simulink model "feedback_lin"  (R2022b)
settings: Solver=ode4  StartTime=0.0  StopTime=t_end  FixedStep=t_step  RelTol=1e-3
undefined symbols (not defined in the file): AW, C, d_delta, d_on, d_time, d_val, E, iL0, K0i, K1i, K_r, Ki, Kif, Kn, Kti, Ku, L, n_on, R, r_delta, r_on, r_sel, r_time, r_val, sel, sigma_n, t_step, uC0, wp, y0
libraries: fuzblock x1
settings Model: Creator=Milosh Yokich  LastModifiedBy=Milosh Yokich
settings SolverCC: AlgebraicLoopSolver=TrustRegion
settings DataIOCC: ReturnWorkspaceOutputs=off
settings DebuggingCC: UnconnectedInputMsg=warning  UnconnectedOutputMsg=warning  UnconnectedLineMsg=warning  SFMachineParentedDataDiag=warning  ArithmeticOperatorsInVariantConditions=warning
settings ModelReferenceCC: EnableRefExpFcnMdlSchedulingChecks=on
settings SFSimCC: SimUseLocalCustomCode=off  CustomCodeUndefinedFunction=UseInterfaceOnly
settings RTWCC: RTWUseLocalCustomCode=off

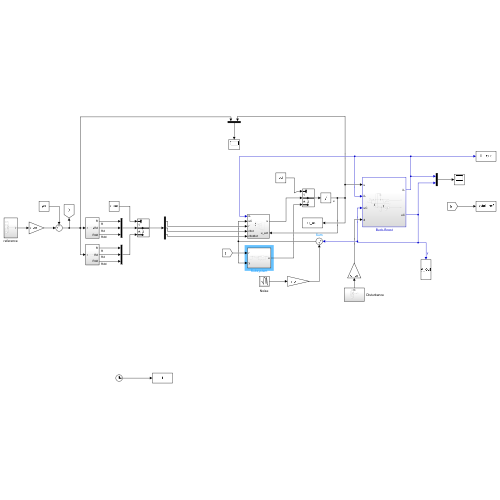
[thumbnail: Simulink's stored preview of the top-level diagram]
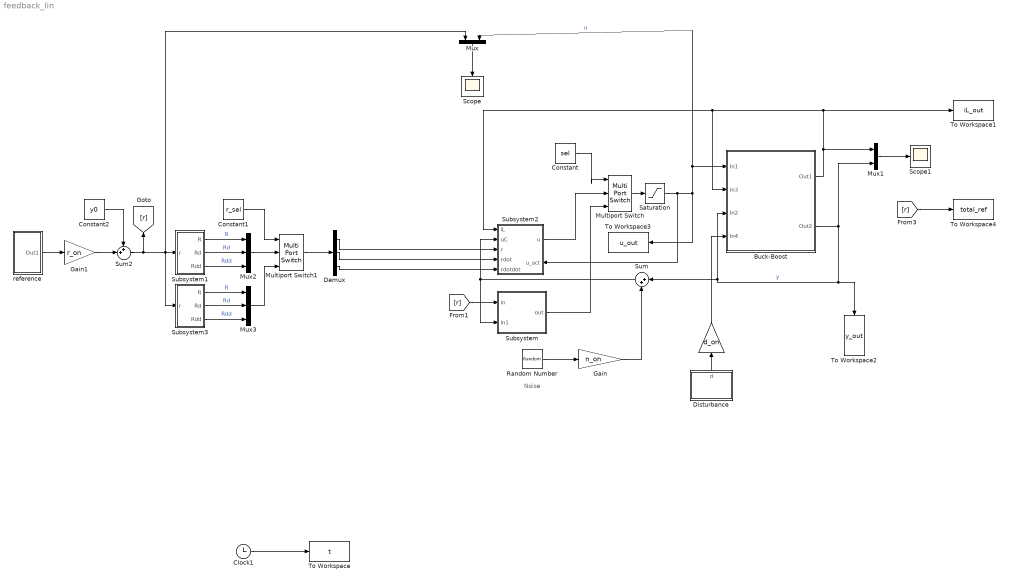
== system feedback_lin ==
  note: Noise
  " " : Gain  Gain=d_on
  Buck-Boost : Subsystem
  Clock1 : Clock
  Constant : Constant  Value=sel
  Constant1 : Constant  Value=r_sel
  Constant2 : Constant  Value=y0
  Demux : Demux  Outputs=3
  Disturbance : Subsystem
  Gain : Gain  Gain=n_on
  Gain1 : Gain  Gain=r_on
  Multiport Switch : MultiPortSwitch  Inputs=2  SaturateOnIntegerOverflow=off  InputSameDT=off
  Multiport Switch1 : MultiPortSwitch  Inputs=2  SaturateOnIntegerOverflow=off  InputSameDT=off
  Mux : Mux  Inputs=2
  Mux1 : Mux  Inputs=2
  Mux2 : Mux  Inputs=3
  Mux3 : Mux  Inputs=3
  Random Number : RandomNumber  Variance=sigma_n  SampleTime=t_step
  Saturation : Saturate  UpperLimit=1  LowerLimit=0
  Scope : Scope
  Scope1 : Scope
  Subsystem : Subsystem
  Subsystem1 : Subsystem
  Subsystem2 : Subsystem
      settings: PortSchema="{\"entries\":[{\"content\":{\"sides\":[{\"content\":{\"connectorIds\":[\"In1\",\"In2\",\"In3\",\"In4\",\"In5\"]},\"type\":\"ConnectorPlacement.EquallySpacedRectSide\",\"uuid\":\"a5ffe97d-c71e-4de0-ba63-bc76db2e4a28\"},{\"content\":{\"connectorIds\":[\"Out1\",\"In6\"],\"side\":\"RIGHT\"},\"type\":\"ConnectorPlacement.EquallySpacedRectSide\",\"uuid\":\"4d46e151-a221-479a-a7c8-fb4e18a057b4\"},{\"content\":{\"connectorIds\":[],\"side\":\"TOP\"},\"type\":\"ConnectorPlacement.EquallySpacedRectSide\",\"uuid\":\"a0b468b3-16b9-437b-958e-968171817142\"},{\"content\":{\"connectorIds\":[],\"side\":\"BOTTOM\"},\"type\":\"ConnectorPlacement.EquallySpacedRectSide\",\"uuid\":\"210b4f3c-ba38-4a79-8d72-0619259306c1\"}]},\"type\":\"ConnectorPlacement.EquallySpacedConnector\",\"uuid\":\"c6942702-5a6a-49ce-9e2c-c5f8d8595752\"}],\"packageUris\":[\"http://schema.mathworks.com/mf0/Connector/R2020b\"],\"version\":\"1.0\"}"
  Subsystem3 : Subsystem
  Sum : Sum  Inputs=|++
  Sum2 : Sum  Inputs=++|
  To Workspace : ToWorkspace  VariableName=t  SampleTime=-1
  To Workspace1 : ToWorkspace  VariableName=iL_out  SampleTime=-1
  To Workspace2 : ToWorkspace  VariableName=y_out  SampleTime=-1
  To Workspace3 : ToWorkspace  VariableName=u_out  SampleTime=-1
  To Workspace4 : ToWorkspace  VariableName=total_ref  SampleTime=-1
  "reference " : Subsystem
  wires:
  Random Number/1 -> Gain/1
  Clock1/1 -> To Workspace/1
  Mux/1 -> Scope/1
  Mux1/1 -> Scope1/1
  Saturation/1 -> Subsystem2/6(u_act), Buck-Boost/1(In1), Mux/2, To Workspace3/1  "u"
  [r] -> To Workspace4/1
  Disturbance/1(d) -> " "/1
  "reference "/1(Out1) -> Gain1/1
  Gain/1 -> Sum/2
  Buck-Boost/2(Out2) -> Buck-Boost/3(In2), Sum/1, To Workspace2/1, Mux1/2  "y"
  Buck-Boost/1(Out1) -> Subsystem2/1(iL), Buck-Boost/2(In3), To Workspace1/1, Mux1/1
  " "/1 -> Buck-Boost/4(In4)
  Constant2/1 -> Sum2/1
  Multiport Switch/1 -> Saturation/1
  Constant/1 -> Multiport Switch/1
  Sum2/1 -> Subsystem3/1(r), Subsystem1/1(r), Mux/1, [r]
  Gain1/1 -> Sum2/2
  Subsystem1/1(R) -> Mux2/1  "R"
  Subsystem1/2(Rd) -> Mux2/2  "Rd"
  Subsystem1/3(Rdd) -> Mux2/3  "Rdd"
  Subsystem3/1(R) -> Mux3/1  "R"
  Subsystem3/2(Rd) -> Mux3/2  "Rd"
  Subsystem3/3(Rdd) -> Mux3/3  "Rdd"
  Mux2/1 -> Multiport Switch1/2
  Mux3/1 -> Multiport Switch1/3
  Constant1/1 -> Multiport Switch1/1
  Multiport Switch1/1 -> Demux/1
  Demux/3 -> Subsystem2/5(rdotdot)
  Demux/2 -> Subsystem2/4(rdot)
  Demux/1 -> Subsystem2/3(r)
  [r] -> Subsystem/1(in)
  Sum/1 -> Subsystem/2(in1), Subsystem2/2(uC)
  Subsystem2/1(u) -> Multiport Switch/2
  Subsystem/1(out) -> Multiport Switch/3

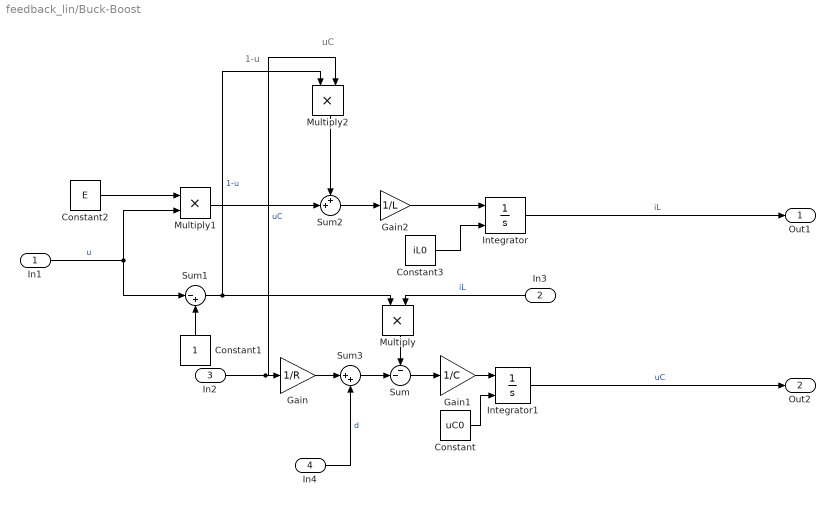
== system feedback_lin/Buck-Boost ==
  note: uC
  note: 1-u
  In1 : Inport
  In3 : Inport  Port=2
  In2 : Inport  Port=3
  In4 : Inport  Port=4
  Constant : Constant  Value=uC0
  Constant1 : Constant
  Constant2 : Constant  Value=E
  Constant3 : Constant  Value=iL0
  Gain : Gain  Gain=1/R
  Gain1 : Gain  Gain=1/C
  Gain2 : Gain  Gain=1/L
  Integrator : Integrator  InitialConditionSource=external
  Integrator1 : Integrator  InitialConditionSource=external
  Multiply : Product
  Multiply1 : Product
  Multiply2 : Product
  Sum : Sum  Inputs=--|
  Sum1 : Sum  Inputs=|-+
  Sum2 : Sum  Inputs=++|
  Sum3 : Sum  Inputs=|++
  Out1 : Outport  VectorParamsAs1DForOutWhenUnconnected=off
  Out2 : Outport  Port=2  VectorParamsAs1DForOutWhenUnconnected=off
  wires:
  In4/1 -> Sum3/2  "d"
  Sum3/1 -> Sum/2
  Gain/1 -> Sum3/1
  In3/1 -> Multiply/2  "iL"
  In2/1 -> Gain/1, Multiply2/2  "uC"
  Sum2/1 -> Gain2/1
  Sum/1 -> Gain1/1
  Constant/1 -> Integrator1/2
  Constant1/1 -> Sum1/2
  Multiply/1 -> Sum/1
  Constant3/1 -> Integrator/2
  In1/1 -> Sum1/1, Multiply1/2  "u"
  Multiply1/1 -> Sum2/2
  Gain1/1 -> Integrator1/1
  Integrator/1 -> Out1/1  "iL"
  Gain2/1 -> Integrator/1
  Sum1/1 -> Multiply2/1, Multiply/1  "1-u"
  Integrator1/1 -> Out2/1  "uC"
  Constant2/1 -> Multiply1/1
  Multiply2/1 -> Sum2/1

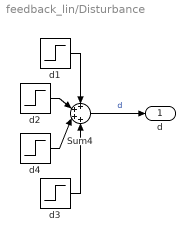
== system feedback_lin/Disturbance ==
  Sum4 : Sum  Inputs=++++
  "d1 " : Step  Time=d_time  After=d_val  SampleTime=0
  "d2 " : Step  Time=d_time + d_delta  After=-d_val  SampleTime=0
  "d3 " : Step  Time=d_time + d_delta*2  After=-d_val  SampleTime=0
  "d4 " : Step  Time=d_time + d_delta*3  After=d_val  SampleTime=0
  d : Outport  VectorParamsAs1DForOutWhenUnconnected=off
  wires:
  "d3 "/1 -> Sum4/4
  "d1 "/1 -> Sum4/1
  "d2 "/1 -> Sum4/2
  "d4 "/1 -> Sum4/3
  Sum4/1 -> d/1  "d"

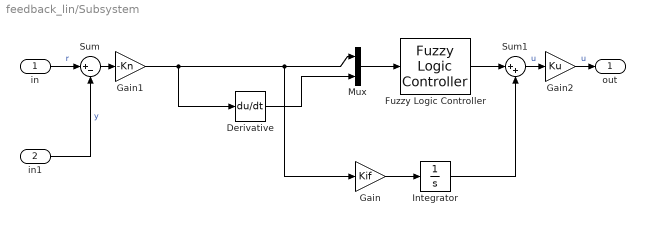
== system feedback_lin/Subsystem ==
  in : Inport
  in1 : Inport  Port=2
  Derivative : Derivative  CoefficientInTFapproximation=1/200
  Fuzzy Logic Controller : fuzblock/Fuzzy Logic  Controller  FIS='pravila.fis'  OutputSampleNumber=101  DataType=double  FuzzifiedInputs=off  RuleFiringStrengths=off  RuleOutputs=off  AggregatedOutputs=off  SimulateUsing=Code generation  OutOfRangeInputValueMessage=none  NoRuleFiredMessage=none  EmptyOutputFuzzySetMessage=none
  Gain : Gain  Gain=Kif
  Gain1 : Gain  Gain=-Kn
  Gain2 : Gain  Gain=Ku
  Integrator : Integrator
  Mux : Mux  Inputs=2
  Sum : Sum  Inputs=|+-
  Sum1 : Sum  Inputs=|++
  out : Outport
  wires:
  in/1 -> Sum/1  "r"
  in1/1 -> Sum/2  "y"
  Sum/1 -> Gain1/1
  Fuzzy Logic Controller/1 -> Sum1/1
  Integrator/1 -> Sum1/2
  Sum1/1 -> Gain2/1  "u"
  Gain/1 -> Integrator/1
  Gain1/1 -> Derivative/1, Gain/1, Mux/1
  Gain2/1 -> out/1  "u"
  Mux/1 -> Fuzzy Logic Controller/1
  Derivative/1 -> Mux/2

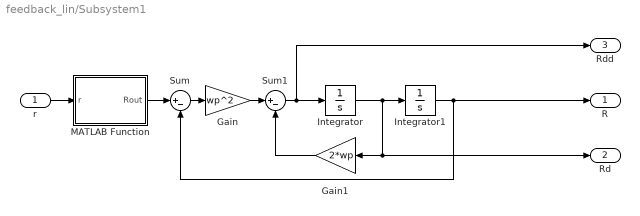
== system feedback_lin/Subsystem1 ==
  r : Inport
  Gain : Gain  Gain=wp^2
  Gain1 : Gain  Gain=2*wp
  Integrator : Integrator
  Integrator1 : Integrator
  MATLAB Function : MATLAB Function  TreatAsAtomicUnit=on
  Sum : Sum  Inputs=|+-
  Sum1 : Sum  Inputs=|+-
  R : Outport
  Rd : Outport  Port=2
  Rdd : Outport  Port=3
  wires:
  r/1 -> MATLAB Function/1(r)
  MATLAB Function/1(Rout) -> Sum/1
  Sum/1 -> Gain/1
  Gain/1 -> Sum1/1
  Sum1/1 -> Rdd/1, Integrator/1
  Gain1/1 -> Sum1/2
  Integrator/1 -> Rd/1, Gain1/1, Integrator1/1
  Integrator1/1 -> Sum/2, R/1

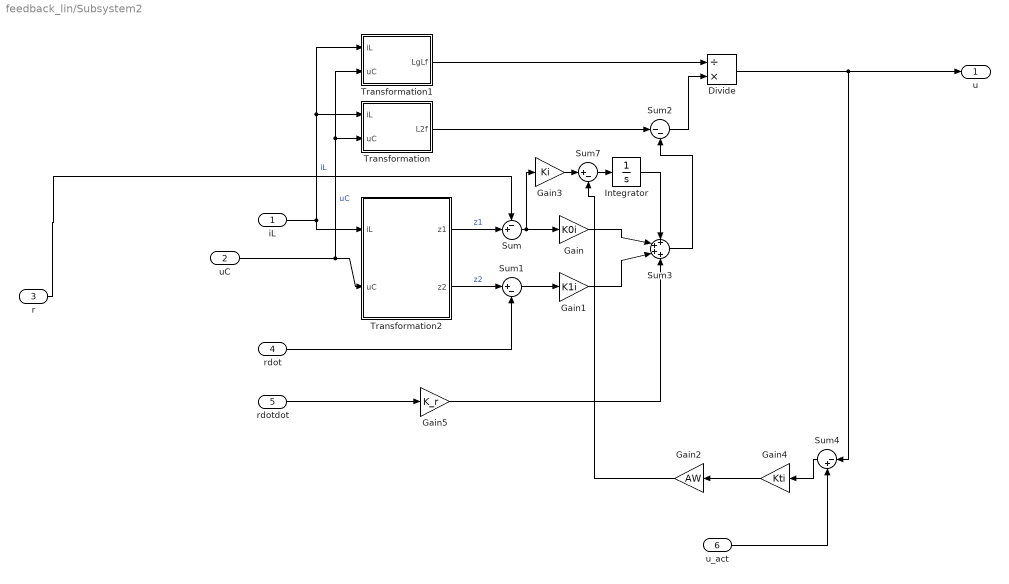
== system feedback_lin/Subsystem2 ==
  iL : Inport
  uC : Inport  Port=2
  r : Inport  Port=3
  rdot : Inport  Port=4
  rdotdot : Inport  Port=5
  u_act : Inport  Port=6
  Divide : Product  Inputs=/*
  Gain : Gain  Gain=K0i
  Gain1 : Gain  Gain=K1i
  Gain2 : Gain  Gain=AW
  Gain3 : Gain  Gain=Ki
  Gain4 : Gain  Gain=Kti
  Gain5 : Gain  Gain=K_r
  Integrator : Integrator  UpperSaturationLimit=30  LowerSaturationLimit=-30
  Sum : Sum  Inputs=-+|
  Sum1 : Sum  Inputs=|+-
  Sum2 : Sum  Inputs=|--
  Sum3 : Sum  Inputs=++++
  Sum4 : Sum  Inputs=|-+
  Sum7 : Sum  Inputs=|+-
  Transformation : MATLAB Function  TreatAsAtomicUnit=on
  Transformation1 : MATLAB Function  TreatAsAtomicUnit=on
  Transformation2 : MATLAB Function  TreatAsAtomicUnit=on
  u : Outport
  wires:
  iL/1 -> Transformation/1(iL), Transformation1/1(iL), Transformation2/1(iL)  "iL"
  Transformation2/1(z1) -> Sum/2  "z1"
  Transformation2/2(z2) -> Sum1/1  "z2"
  uC/1 -> Transformation1/2(uC), Transformation/2(uC), Transformation2/2(uC)  "uC"
  Sum/1 -> Gain/1, Gain3/1
  Sum1/1 -> Gain1/1
  Transformation/1(L2f) -> Sum2/1
  Transformation1/1(LgLf) -> Divide/1
  Sum2/1 -> Divide/2
  Divide/1 -> Sum4/1, u/1
  Sum4/1 -> Gain4/1
  u_act/1 -> Sum4/2
  Gain4/1 -> Gain2/1
  Gain3/1 -> Sum7/1
  Sum7/1 -> Integrator/1
  Integrator/1 -> Sum3/1
  Gain/1 -> Sum3/2
  Gain1/1 -> Sum3/3
  Sum3/1 -> Sum2/2
  Gain2/1 -> Sum7/2
  r/1 -> Sum/1
  rdotdot/1 -> Gain5/1
  Gain5/1 -> Sum3/4
  rdot/1 -> Sum1/2

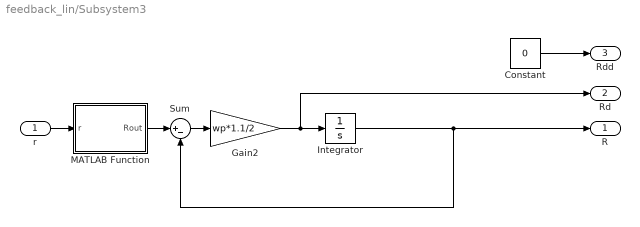
== system feedback_lin/Subsystem3 ==
  r : Inport
  Constant : Constant  Value=0
  Gain2 : Gain  Gain=wp*1.1/2
  Integrator : Integrator
  MATLAB Function : MATLAB Function  TreatAsAtomicUnit=on
  Sum : Sum  Inputs=|+-
  R : Outport
  Rd : Outport  Port=2
  Rdd : Outport  Port=3
  wires:
  r/1 -> MATLAB Function/1(r)
  MATLAB Function/1(Rout) -> Sum/1
  Sum/1 -> Gain2/1
  Gain2/1 -> Rd/1, Integrator/1
  Integrator/1 -> Sum/2, R/1
  Constant/1 -> Rdd/1

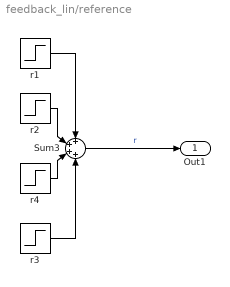
== system feedback_lin/reference  ==
  Sum3 : Sum  Inputs=++++
  "r1 " : Step  Time=r_time  After=r_val  SampleTime=0
  "r2 " : Step  Time=r_time + r_delta  After=-r_val  SampleTime=0
  "r3 " : Step  Time=r_time + 2*r_delta  After=-r_val  SampleTime=0
  "r4 " : Step  Time=r_time + 3*r_delta  After=r_val  SampleTime=0
  Out1 : Outport  VectorParamsAs1DForOutWhenUnconnected=off
  wires:
  Sum3/1 -> Out1/1  "r"
  "r2 "/1 -> Sum3/2
  "r3 "/1 -> Sum3/4
  "r4 "/1 -> Sum3/3
  "r1 "/1 -> Sum3/1

== matlab function feedback_lin/Subsystem1/MATLAB Function ==
  data: r input; Rout output
function Rout = convert(r)

E = 12; %V
R = 52; %Omh
L = 0.01591; %H
C = 0.000470; %F 


Vc = -22.5;
uCe = Vc;
ue = -(uCe)/(E-uCe);
iLe = -uCe/R/(1-ue);

uC = r;
u = -(uC)/(E-uC);
iL = -uC/R/(1-u);


gamma = L*1/2*iLe^2 + C*1/2*(uCe - E)^2;
gamma = -gamma;

Rout = L*1/2*iL^2 + C*1/2*(uC - E)^2 + gamma;

== matlab function feedback_lin/Subsystem2/Transformation ==
  data: iL input; L2f output; uC input
function L2f = L2f(iL, uC)
E = 12; %V
R = 52; %Omh
L = 0.01591; %H
C = 0.000470; %F 

L2f = E/L*uC - 1/(R*C)*(iL + uC/R)*(-2*uC + E);

== matlab function feedback_lin/Subsystem2/Transformation1 ==
  data: iL input; LgLf output; uC input
function LgLf = LgLf(iL, uC)
E = 12; %V
R = 52; %Omh
L = 0.01591; %H
C = 0.000470; %F 

LgLf = E/L*(-uC + E) + 1/(C*R)*iL*(-2*uC + E);

== matlab function feedback_lin/Subsystem2/Transformation2 ==
  data: iL input; z1 output; uC input; z2 output
function [z1, z2] = T(iL, uC)
E = 12; %V
R = 52; %Omh
L = 0.01591; %H
C = 0.000470; %F 

Vc = -22.5;
uCe = Vc;
ue = -(uCe)/(E-uCe);
iLe = -uCe/R/(1-ue);

gamma = L*1/2*iLe^2 + C*1/2*(uCe - E)^2;
gamma = -gamma;


% z1 = h(x)
z1 = L*1/2*iL^2 + C*1/2*(uC - E)^2 + gamma;
% z2 = Lf h(x)
z2 = E*(iL + uC/R) - uC^2/R;

== matlab function feedback_lin/Subsystem3/MATLAB Function ==
  data: r input; Rout output
function Rout = convert(r)

E = 12; %V
R = 52; %Omh
L = 0.01591; %H
C = 0.000470; %F 


Vc = -22.5;
uCe = Vc;
ue = -(uCe)/(E-uCe);
iLe = -uCe/R/(1-ue);

uC = r;
u = -(uC)/(E-uC);
iL = -uC/R/(1-u);


gamma = L*1/2*iLe^2 + C*1/2*(uCe - E)^2;
gamma = -gamma;

Rout = L*1/2*iL^2 + C*1/2*(uC - E)^2 + gamma;
